simulink model "WorkshopB_1v2"  (R2016b)
settings: Solver=ode45  StartTime=0.0  StopTime=1  RelTol=1e-3
values from neighbouring files (symbols this model uses):
  dm = dm*eps_dm    (= 1.3528e-05)    [param.m]
  Dpos = double(D)    [param.m]
  Fc = 0.0013    [param.m]
  Ipos = double(I)    [param.m]
  Jeq = eps_Jeq*Jeq    (= 2.20476e-05)    [param.m]
  Kemf = 1/(137*2*pi/60)    (= 0.0697028947848)    [param.m]
  Km = 69.7E-3    (= 0.0697)    [param.m]
  Max_Accel = Max_torque/Jeq    (= 1356.15667919)    [param.m]
  Max_Speed = 24/Kemf    (= 344.318554833)    [param.m]
  Npos = double(N)    [param.m]
  Ppos = double(P)    [param.m]
  R = s*s + s*N    [PID_calc.m]    (also in param.m = 112)
undefined symbols (not defined in the file or in its folder): sigbuilder_block
settings Model: Creator=sofianh  LastModifiedBy=Philipp
settings DataIOCC: LimitDataPoints=on  SaveFormat=Array
settings OptimizationCC: BlockReduction=off  BooleanDataType=off  LifeSpan=inf
settings DebuggingCC: SaveWithParameterizedLinksMsg=none  UnderspecifiedInitializationDetection=Classic  MergeDetectMultiDrivingBlocksExec=none  SignalResolutionControl=TryResolveAllWithWarning  SFUnexpectedBacktrackingDiag=warning  SFNoUnconditionalDefaultTransitionDiag=warning  SFExecutionAtInitializationDiag=none
settings HardwareCC: ProdBitPerPointer=32  ProdBitPerSizeT=32  ProdBitPerPtrDiffT=32  ProdLargestAtomicFloat=None  ProdIntDivRoundTo=Undefined  ProdEndianess=Unspecified  ProdWordSize=32  ProdHWDeviceType=32-bit Generic  TargetUnknown=on
settings ModelReferenceCC: PropagateSignalLabelsOutOfModel=off
settings GRTTargetCC: TargetLangStandard=C89/C90 (ANSI)  GeneratePreprocessorConditionals=Disable all
settings ConfigComp: CovMetricSettings=dw  CovHtmlReporting=on  CovSaveCumulativeToWorkspaceVar=on  CovSaveSingleToWorkspaceVar=on  CovExternalEMLEnable=off  CovSFcnEnable=off

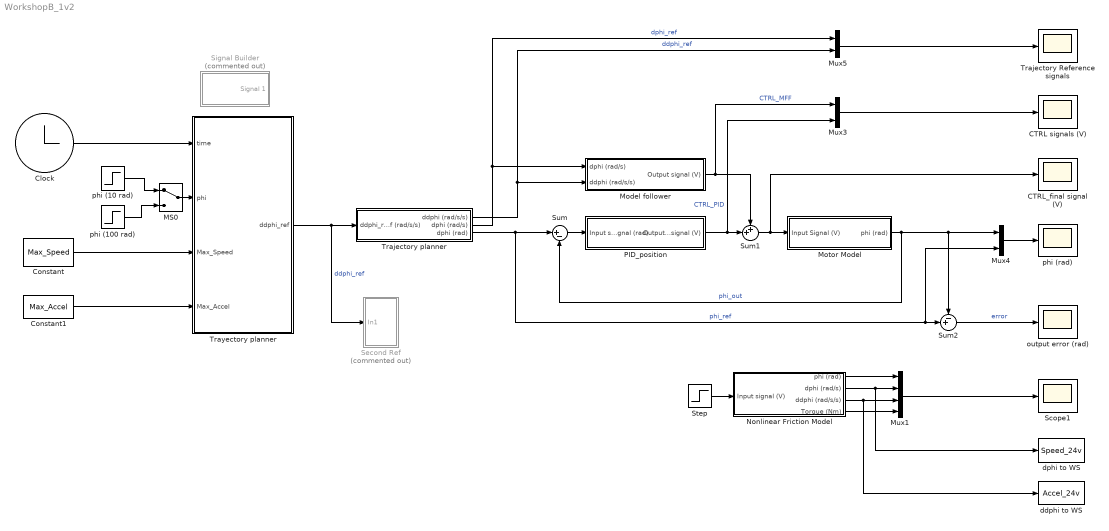
== system WorkshopB_1v2 ==
  CTRL signals (V) : Scope
  CTRL_final signal (V) : Scope
  Clock : Clock
  Constant : Constant  Value=Max_Speed
  Constant1 : Constant  Value=Max_Accel
  MS0 : ManualSwitch
  Model follower : Subsystem
  Motor Model : Subsystem
  Mux1 : Mux
  Mux3 : Mux  Inputs=2
  Mux4 : Mux  Inputs=2
  Mux5 : Mux  Inputs=2
  Nonlinear Friction Model : Subsystem
  PID_position : Subsystem
  Scope1 : Scope
  Second Ref : Subsystem  Commented=on
  Signal Builder : Subsystem  Tag=STV Subsys  Commented=on  LoadFcn=sigbuilder_block('load');  StartFcn=sigbuilder_block('start');  StopFcn=sigbuilder_block('stop');  ClipboardFcn=sigbuilder_block('clipboard');  mask(Sigbuilder block){tuvar=[0:10]}
      mask help: Simulink:masks:SigbuilderBlock_MD
      mask init:
      | if ~strcmp(get_param(bdroot(gcbh),'SimulationStatus'),'stopped') tuvar = sigbuilder_block('maskInit'); end
      settings: CopyFcn=sigbuilder_block('copy');  DeleteFcn=sigbuilder_block('delete');  ModelCloseFcn=sigbuilder_block('modelClose');  PreSaveFcn=sigbuilder_block('preSave');  PauseFcn=sigbuilder_block('pause');  ContinueFcn=sigbuilder_block('continue');  NameChangeFcn=sigbuilder_block('namechange');  OpenFcn=sigbuilder_block('open',[437.6 199.2 550.4 400 ]);  CloseFcn=sigbuilder_block('close');
      mask Display: plot(0, 0, 100, 100,[2, 2, 32, 32, 2], [68, 8, 8, 68, 68],[32, 2], [38, 38], [32, 19, 2],[53, 60, 44], [32, 17, 17, 2],[16, 16, 31, 31]);txt = getActiveGroup(gcbh);text(2, 100, txt,'verticalAlignment', 'top');
  Step : Step  Time=0  After=24  SampleTime=0
  Sum : Sum  Inputs=|+-
  Sum1 : Sum  Inputs=++|
  Sum2 : Sum  Inputs=-+|
  Trajectory Reference signals : Scope
  Trajectory planner : Subsystem
  Trayectory planner : MATLAB Function  TreatAsAtomicUnit=on  SystemSampleTime=1e-3
  ddphi to WS : ToWorkspace  VariableName=Accel_24v  SaveFormat=Timeseries  SampleTime=-1
  dphi to WS : ToWorkspace  VariableName=Speed_24v  SaveFormat=Timeseries  SampleTime=-1
  output error (rad) : Scope
  phi (rad) : Scope
  phi (10 rad) : Step  Time=0  After=10  SampleTime=0
  phi (100 rad) : Step  Time=0  After=100  SampleTime=0
  wires:
  Mux1/1 -> Scope1/1
  Nonlinear Friction Model/1(phi (rad)) -> Mux1/1
  Step/1 -> Nonlinear Friction Model/1(Input signal (V))
  Nonlinear Friction Model/2(dphi (rad/s)) -> dphi to WS/1, Mux1/2
  Nonlinear Friction Model/3(ddphi (rad/s/s)) -> ddphi to WS/1, Mux1/3
  Nonlinear Friction Model/4(Torque (Nm)) -> Mux1/4
  Clock/1 -> Trayectory planner/1(time)
  phi (10 rad)/1 -> MS0/1
  phi (100 rad)/1 -> MS0/2
  MS0/1 -> Trayectory planner/2(phi)
  Constant/1 -> Trayectory planner/3(Max_Speed)
  Constant1/1 -> Trayectory planner/4(Max_Accel)
  Sum/1 -> PID_position/1(Input signal (rad))
  Motor Model/1(phi (rad)) -> Mux4/1, Sum2/1, Sum/2  "phi_out"
  PID_position/1(Output signal (V)) -> Sum1/2, Mux3/2  "CTRL_PID"
  Mux3/1 -> CTRL signals (V)/1
  Model follower/1(Output signal (V)) -> Mux3/1, Sum1/1  "CTRL_MFF"
  Trayectory planner/1(ddphi_ref) -> Second Ref/1(In1), Trajectory planner/1(ddphi_ref (rad/s/s))  "ddphi_ref"
  Mux4/1 -> phi (rad)/1
  Trajectory planner/3(dphi (rad)) -> Sum/1, Mux4/2, Sum2/2  "phi_ref"
  Sum1/1 -> CTRL_final signal (V)/1, Motor Model/1(Input Signal (V))
  Trajectory planner/1(ddphi (rad/s/s)) -> Mux5/2, Model follower/2(ddphi (rad/s/s))  "ddphi_ref"
  Mux5/1 -> Trajectory Reference signals/1
  Trajectory planner/2(dphi (rad/s)) -> Mux5/1, Model follower/1(dphi (rad/s))  "dphi_ref"
  Sum2/1 -> output error (rad)/1  "error"

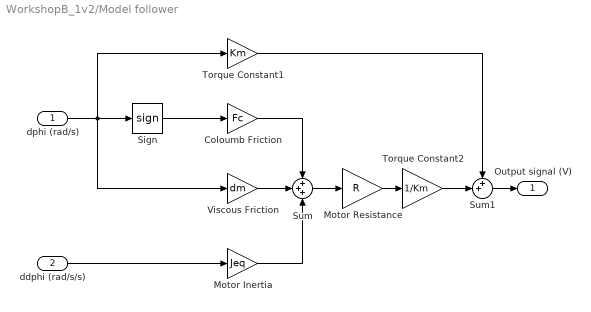
== system WorkshopB_1v2/Model follower ==
  dphi (rad/s) : Inport
  ddphi (rad/s/s) : Inport  Port=2
  Coloumb Friction : Gain  Gain=Fc
  "Motor Inertia " : Gain  Gain=Jeq
  Motor Resistance : Gain  Gain=R
  Sign : Signum
  Sum : Sum  Inputs=+++
  Sum1 : Sum  Inputs=++|
  Torque Constant1 : Gain  Gain=Km
  Torque Constant2 : Gain  Gain=1/Km
  Viscous Friction : Gain  Gain=dm
  Output signal (V) : Outport
  wires:
  ddphi (rad/s/s)/1 -> "Motor Inertia "/1
  dphi (rad/s)/1 -> Viscous Friction/1, Torque Constant1/1, Sign/1
  "Motor Inertia "/1 -> Sum/3
  Viscous Friction/1 -> Sum/2
  Sum/1 -> Motor Resistance/1
  Torque Constant1/1 -> Sum1/1
  Motor Resistance/1 -> Torque Constant2/1
  Sum1/1 -> Output signal (V)/1
  Sign/1 -> Coloumb Friction/1
  Coloumb Friction/1 -> Sum/1
  Torque Constant2/1 -> Sum1/2

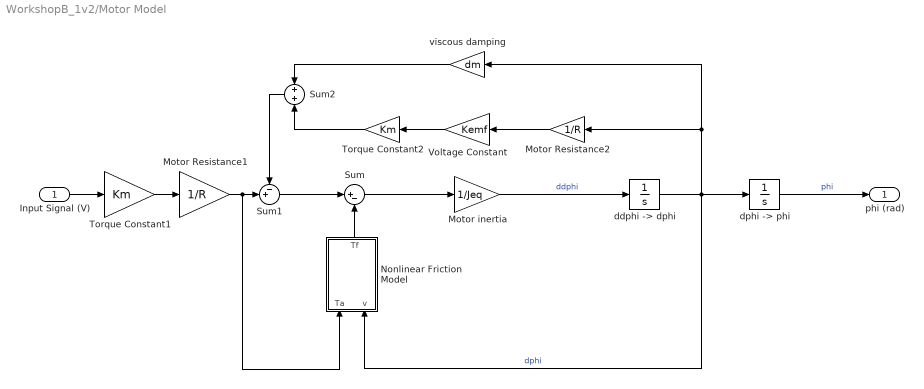
== system WorkshopB_1v2/Motor Model ==
  Input Signal (V) : Inport
  Motor Resistance1 : Gain  Gain=1/R
  Motor Resistance2 : Gain  Gain=1/R
  Motor inertia : Gain  Gain=1/Jeq
  Nonlinear Friction Model : MATLAB Function  TreatAsAtomicUnit=on
  Sum : Sum  Inputs=|+-
  Sum1 : Sum  Inputs=-+|
  Sum2 : Sum  Inputs=+|+
  Torque Constant1 : Gain  Gain=Km
  Torque Constant2 : Gain  Gain=Km
  Voltage Constant : Gain  Gain=Kemf
  "ddphi -> dphi" : Integrator
  "dphi -> phi" : Integrator
  viscous damping : Gain  Gain=dm
  phi (rad) : Outport
  wires:
  Motor Resistance1/1 -> Nonlinear Friction Model/1(Ta), Sum1/2
  Sum2/1 -> Sum1/1
  "ddphi -> dphi"/1 -> Nonlinear Friction Model/2(v), "dphi -> phi"/1, viscous damping/1, Motor Resistance2/1  "dphi"
  Sum/1 -> Motor inertia/1
  Sum1/1 -> Sum/1
  Nonlinear Friction Model/1(Tf) -> Sum/2
  "dphi -> phi"/1 -> phi (rad)/1  "phi"
  Motor inertia/1 -> "ddphi -> dphi"/1  "ddphi"
  Torque Constant1/1 -> Motor Resistance1/1
  Voltage Constant/1 -> Torque Constant2/1
  viscous damping/1 -> Sum2/1
  Torque Constant2/1 -> Sum2/2
  Motor Resistance2/1 -> Voltage Constant/1
  Input Signal (V)/1 -> Torque Constant1/1

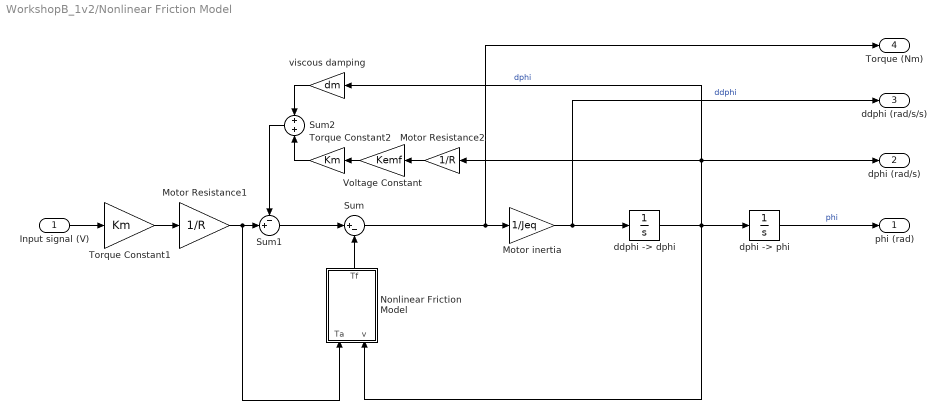
== system WorkshopB_1v2/Nonlinear Friction Model ==
  Input signal (V) : Inport
  Motor Resistance1 : Gain  Gain=1/R
  Motor Resistance2 : Gain  Gain=1/R
  Motor inertia : Gain  Gain=1/Jeq
  Nonlinear Friction Model : MATLAB Function  TreatAsAtomicUnit=on
  Sum : Sum  Inputs=|+-
  Sum1 : Sum  Inputs=-+|
  Sum2 : Sum  Inputs=+|+
  Torque Constant1 : Gain  Gain=Km
  Torque Constant2 : Gain  Gain=Km
  Voltage Constant : Gain  Gain=Kemf
  "ddphi -> dphi" : Integrator
  "dphi -> phi" : Integrator
  viscous damping : Gain  Gain=dm
  phi (rad) : Outport
  dphi (rad/s) : Outport  Port=2
  ddphi (rad/s/s) : Outport  Port=3
  Torque (Nm) : Outport  Port=4
  wires:
  Motor Resistance1/1 -> Nonlinear Friction Model/1(Ta), Sum1/2
  Sum2/1 -> Sum1/1
  "ddphi -> dphi"/1 -> Nonlinear Friction Model/2(v), "dphi -> phi"/1, viscous damping/1, Motor Resistance2/1, dphi (rad/s)/1  "dphi"
  Input signal (V)/1 -> Torque Constant1/1
  Sum/1 -> Torque (Nm)/1, Motor inertia/1
  Sum1/1 -> Sum/1
  Nonlinear Friction Model/1(Tf) -> Sum/2
  "dphi -> phi"/1 -> phi (rad)/1  "phi"
  Motor inertia/1 -> "ddphi -> dphi"/1, ddphi (rad/s/s)/1  "ddphi"
  Torque Constant1/1 -> Motor Resistance1/1
  Voltage Constant/1 -> Torque Constant2/1
  viscous damping/1 -> Sum2/1
  Torque Constant2/1 -> Sum2/2
  Motor Resistance2/1 -> Voltage Constant/1

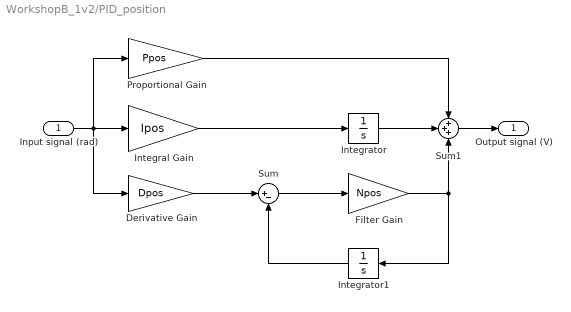
== system WorkshopB_1v2/PID_position ==
  Input signal (rad) : Inport
  Derivative Gain : Gain  Gain=Dpos
  Filter Gain : Gain  Gain=Npos
  Integral Gain : Gain  Gain=Ipos
  Integrator : Integrator
  Integrator1 : Integrator
  Proportional Gain : Gain  Gain=Ppos
  Sum : Sum  Inputs=|+-
  Sum1 : Sum  Inputs=+++
  Output signal (V) : Outport
  wires:
  Sum1/1 -> Output signal (V)/1
  Integrator/1 -> Sum1/2
  Integrator1/1 -> Sum/2
  Filter Gain/1 -> Sum1/3, Integrator1/1
  Sum/1 -> Filter Gain/1
  Derivative Gain/1 -> Sum/1
  Integral Gain/1 -> Integrator/1
  Proportional Gain/1 -> Sum1/1
  Input signal (rad)/1 -> Derivative Gain/1, Integral Gain/1, Proportional Gain/1

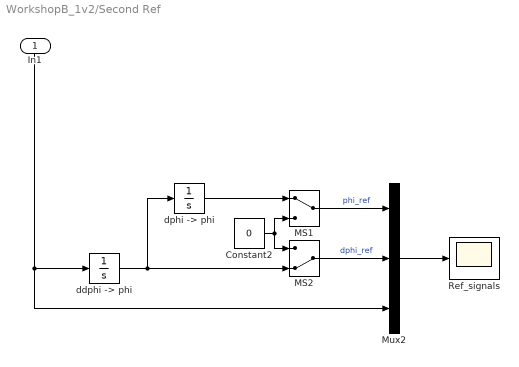
== system WorkshopB_1v2/Second Ref ==
  In1 : Inport
  Constant2 : Constant  Value=0
  MS1 : ManualSwitch
  MS2 : ManualSwitch  CurrentSetting=0
  Mux2 : Mux  Inputs=3
  Ref_signals : Scope
  "ddphi -> phi" : Integrator
  "dphi -> phi" : Integrator
  wires:
  "ddphi -> phi"/1 -> "dphi -> phi"/1, MS2/2
  Mux2/1 -> Ref_signals/1
  MS1/1 -> Mux2/1  "phi_ref"
  Constant2/1 -> MS2/1, MS1/2
  MS2/1 -> Mux2/2  "dphi_ref"
  In1/1 -> Mux2/3, "ddphi -> phi"/1
  "dphi -> phi"/1 -> MS1/1

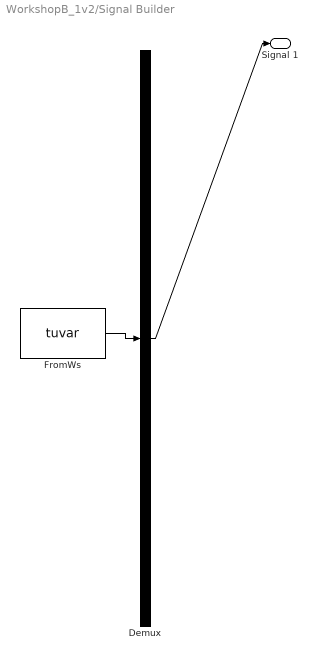
== system WorkshopB_1v2/Signal Builder ==
  Demux : Demux  Tag=STV Demux  Outputs=1
  FromWs : FromWorkspace  Tag=STV FromWs  VariableName=tuvar  SampleTime=0
      SigBuilderData=|
      | common.afterFinalStr = 'Extrapolate'
      | common.sampleTime = 0
      | dataSet.timeRange = [0 1]
      | dataSet.name = 'Group 1'
      | sbobj.Groups.Name = 'Group 1'
      | sbobj.Groups.Signals.Name = 'Signal 1'
      | sbobj.Groups.Signals.XData = [0 0.253892901991 0.253892901991 0.507785803983 0.507785803983 1]
      | sbobj.Groups.Signals.YData = [100 100 -100 -100 0 0]
      | sbobj.Groups.TimeRange = [0 1]
  Signal 1 : Outport  Tag=STV Outport
  wires:
  FromWs/1 -> Demux/1
  Demux/1 -> Signal 1/1

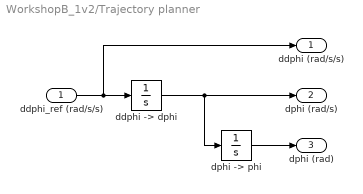
== system WorkshopB_1v2/Trajectory planner ==
  ddphi_ref (rad/s/s) : Inport
  "ddphi -> dphi" : Integrator
  "dphi -> phi" : Integrator
  ddphi (rad/s/s) : Outport
  dphi (rad/s) : Outport  Port=2
  dphi (rad) : Outport  Port=3
  wires:
  "ddphi -> dphi"/1 -> "dphi -> phi"/1, dphi (rad/s)/1
  ddphi_ref (rad/s/s)/1 -> "ddphi -> dphi"/1, ddphi (rad/s/s)/1
  "dphi -> phi"/1 -> dphi (rad)/1

== matlab function WorkshopB_1v2/Trayectory planner ==
  data: time input; ddphi_ref output; phi input; Max_Speed input; Max_Accel input
function ddphi_ref = Planner(time,phi,Max_Speed, Max_Accel)

trising = Max_Speed/Max_Accel;
Pos_rising = trising*0.5*Max_Speed;
if 2*Pos_rising > phi
    trising = sqrt(phi/Max_Accel);
    if time < trising
        ddphi_ref = Max_Accel;
    elseif time >= trising && time < 2*trising
        ddphi_ref = - Max_Accel;
    else
        ddphi_ref = 0;
    end
else
    t_est = (phi - Max_Speed*trising)/Max_Speed;
    if time < trising
        ddphi_ref = Max_Accel;
    elseif time >= trising && time < (trising + t_est)
        ddphi_ref = 0; 
    elseif time >= (trising + t_est) && time < (2*trising + t_est)
        ddphi_ref = - Max_Accel;
    else
        ddphi_ref = 0;
    end
end

== matlab function WorkshopB_1v2/Nonlinear Friction Model/Nonlinear Friction Model ==
  data: Ta input; v input; Tf output
function Tf = fcn(Ta,v)
Tc = 1e-3;
dv = 1e-1;
if abs(v) < dv
    if abs(Ta) > Tc
        Tf = Tc*sign(Ta);
    else
        Tf = Ta;
    end
else
    Tf = Tc*sign(v);
end

== matlab function WorkshopB_1v2/Motor Model/Nonlinear Friction Model ==
  data: Ta input; v input; Tf output
function Tf = fcn(Ta,v)
Tc = 1e-3;
dv = 1e-1;
if abs(v) < dv
    if abs(Ta) > Tc
        Tf = Tc*sign(Ta);
    else
        Tf = Ta;
    end
else
    Tf = Tc*sign(v);
end
